simulink library "mySLLib"  (R2025a)
settings: Solver=VariableStepAuto  StartTime=0.0  StopTime=10.0  RelTol=1e-3
undefined symbols (not defined in the file or in its folder): ctrl_KPi, ctrl_Tsample
libraries: simulink x1, libKollege x1
settings Model: Creator=jonat  LastModifiedBy=jonat

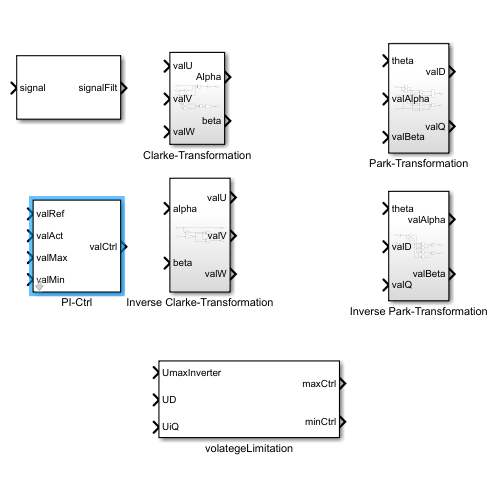
[thumbnail: Simulink's stored preview of the top-level diagram]
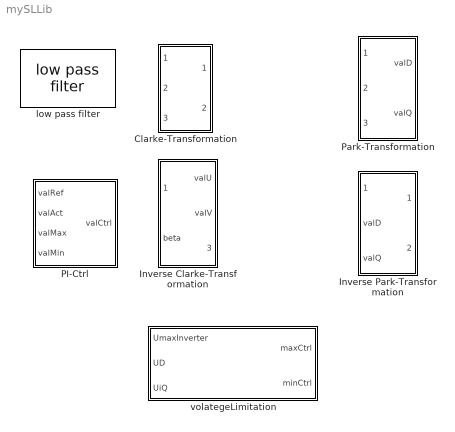
== system mySLLib ==
  Clarke-Transformation : Subsystem
  Inverse Clarke-Transformation : Subsystem
  Inverse Park-Transformation : Subsystem
  PI-Ctrl : Subsystem  mask{localGain=ctrl_KPi, localTsample=ctrl_Tsample, localKi=0}
      mask prompts: localGain "Proportionalfaktor Kp"; localTsample "Abtastzeit (s)"; localKi "Intergralfaktor Ki"
      mask help: Dieser Block implementiert einen zeitdiskreten PI-Regler mit Anti-Wind-up-Funktionalitaet.
      mask DialogControl ParameterGroupVar Prompt: Reglerparameter
  Park-Transformation : Subsystem
  low pass filter : libKollege/low pass filter  localTFilt=1  localTsample=1
  volategeLimitation : Subsystem
      mask help: Berechnung der maximalen Q-Spannung aufgrund der begrenzten Umrichterausgangsspannung.

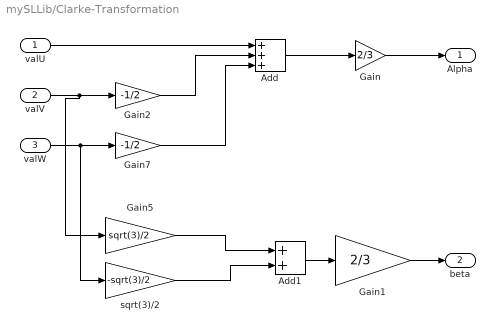
== system mySLLib/Clarke-Transformation ==
  valU : Inport
  valV : Inport  Port=2
  valW : Inport  Port=3
  Add : Sum  Inputs=+++
  Add1 : Sum
  Gain : Gain  Gain=2/3  OutDataTypeStr=single
  Gain1 : Gain  Gain=2/3  OutDataTypeStr=single
  Gain2 : Gain  Gain=-1/2
  Gain5 : Gain  Gain=sqrt(3)/2
  Gain7 : Gain  Gain=-1/2
  sqrt(3)/2 : Gain  Gain=-sqrt(3)/2
  Alpha : Outport
  beta : Outport  Port=2
  wires:
  Gain2/1 -> Add/2
  Gain5/1 -> Add1/1
  Gain1/1 -> beta/1
  sqrt(3)/2/1 -> Add1/2
  Add1/1 -> Gain1/1
  Gain7/1 -> Add/3
  Gain/1 -> Alpha/1
  valU/1 -> Add/1
  valW/1 -> sqrt(3)/2/1, Gain7/1
  Add/1 -> Gain/1
  valV/1 -> Gain2/1, Gain5/1

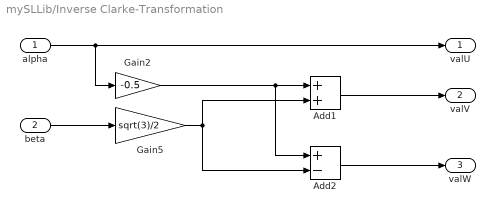
== system mySLLib/Inverse Clarke-Transformation ==
  alpha : Inport
  beta : Inport  Port=2
  Add1 : Sum
  Add2 : Sum  Inputs=+-
  Gain2 : Gain  Gain=-0.5
  Gain5 : Gain  Gain=sqrt(3)/2
  valU : Outport
  valV : Outport  Port=2
  valW : Outport  Port=3
  wires:
  Gain5/1 -> Add2/2, Add1/2
  Add2/1 -> valW/1
  Add1/1 -> valV/1
  Gain2/1 -> Add2/1, Add1/1
  beta/1 -> Gain5/1
  alpha/1 -> valU/1, Gain2/1

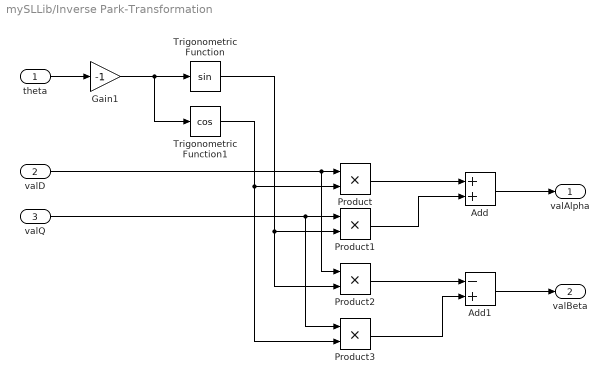
== system mySLLib/Inverse Park-Transformation ==
  theta : Inport
  valD : Inport  Port=2
  valQ : Inport  Port=3
  Add : Sum
  Add1 : Sum  Inputs=-+
  Gain1 : Gain  Gain=-1
  Product{,1..3} (4 alike) : Product
  Trigonometric Function : Trigonometry  OutputSignalType=real
  Trigonometric Function1 : Trigonometry  Operator=cos  OutputSignalType=real
  valAlpha : Outport
  valBeta : Outport  Port=2
  wires:
  Product3/1 -> Add1/2
  Product2/1 -> Add1/1
  Trigonometric Function/1 -> Product1/2, Product2/2
  Product1/1 -> Add/2
  Product/1 -> Add/1
  valQ/1 -> Product3/1, Product1/1
  Trigonometric Function1/1 -> Product/2, Product3/2
  valD/1 -> Product/1, Product2/1
  Gain1/1 -> Trigonometric Function/1, Trigonometric Function1/1
  Add1/1 -> valBeta/1
  Add/1 -> valAlpha/1
  theta/1 -> Gain1/1

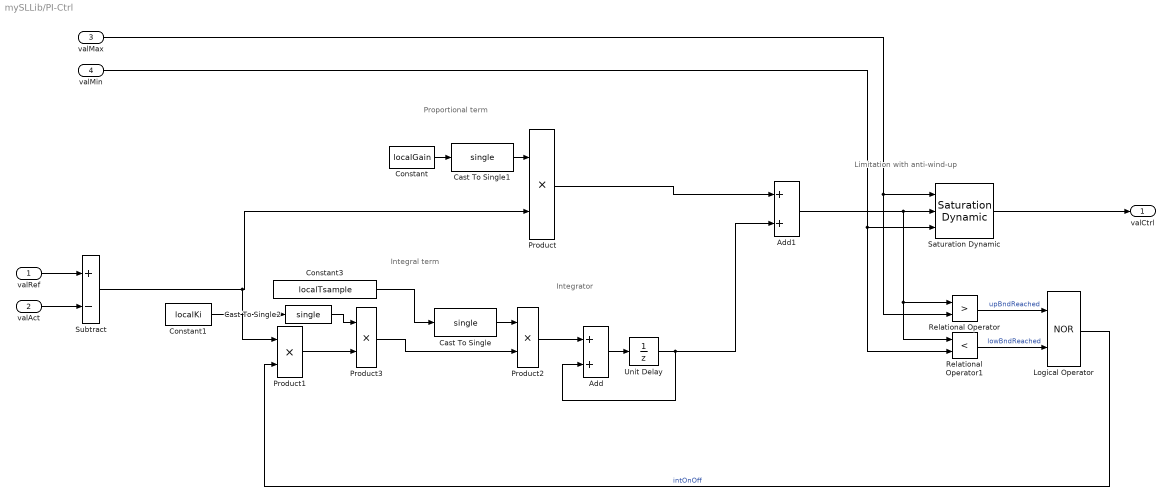
== system mySLLib/PI-Ctrl ==
  note: Integral term
  note: Integrator
  note: Limitation with anti-wind-up
  note: Proportional term
  valRef : Inport
  valAct : Inport  Port=2
  valMax : Inport  Port=3
  valMin : Inport  Port=4
  Add : Sum
  Add1 : Sum
  Cast To Single : DataTypeConversion  OutDataTypeStr=single  SaturateOnIntegerOverflow=off  RndMeth=Floor
  Cast To Single1 : DataTypeConversion  OutDataTypeStr=single  SaturateOnIntegerOverflow=off  RndMeth=Floor
  Cast To Single2 : DataTypeConversion  OutDataTypeStr=single  SaturateOnIntegerOverflow=off  RndMeth=Floor
  Constant : Constant  Value=localGain
  Constant1 : Constant  Value=localKi
  Constant3 : Constant  Value=localTsample
  Logical Operator : Logic  Operator=NOR  AllPortsSameDT=off  OutDataTypeStr=boolean
  Product{,1..3} (4 alike) : Product
  Relational Operator : RelationalOperator  Operator=>  OutDataTypeStr=boolean  InputSameDT=off
  Relational Operator1 : RelationalOperator  Operator=<  OutDataTypeStr=boolean  InputSameDT=off
  Saturation Dynamic : simulink/Discontinuities/Saturation Dynamic  OutMin=[]  OutMax=[]  OutDataTypeStr=Inherit: Same as second input  OutDataType=fixdt(1, 16)  OutScaling=2^-10  DoSatur=off
  Subtract : Sum  Inputs=+-
  Unit Delay : UnitDelay  SampleTime=-1  HasFrameUpgradeWarning=on
  valCtrl : Outport
  wires:
  Add/1 -> Unit Delay/1
  valMin/1 -> Relational Operator1/2, Saturation Dynamic/3
  Logical Operator/1 -> Product1/2  "intOnOff"
  Add1/1 -> Saturation Dynamic/2, Relational Operator/1, Relational Operator1/1
  Product/1 -> Add1/1
  Relational Operator1/1 -> Logical Operator/2  "lowBndReached"
  Constant3/1 -> Cast To Single/1
  valMax/1 -> Saturation Dynamic/1, Relational Operator/2
  Product1/1 -> Product3/2
  Constant/1 -> Cast To Single1/1
  Saturation Dynamic/1 -> valCtrl/1
  valAct/1 -> Subtract/2
  Relational Operator/1 -> Logical Operator/1  "upBndReached"
  Subtract/1 -> Product1/1, Product/2
  valRef/1 -> Subtract/1
  Unit Delay/1 -> Add/2, Add1/2
  Product2/1 -> Add/1
  Cast To Single/1 -> Product2/1
  Cast To Single1/1 -> Product/1
  Product3/1 -> Product2/2
  Cast To Single2/1 -> Product3/1
  Constant1/1 -> Cast To Single2/1

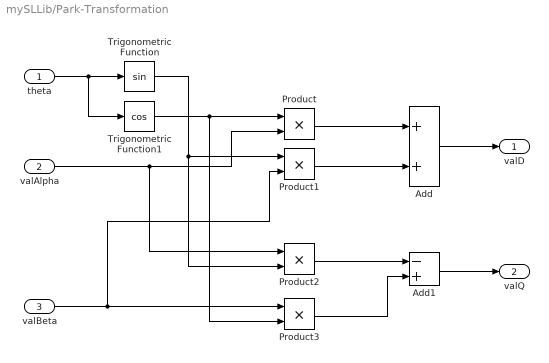
== system mySLLib/Park-Transformation ==
  theta : Inport
  valAlpha : Inport  Port=2
  valBeta : Inport  Port=3
  Add : Sum
  Add1 : Sum  Inputs=-+
  Product{,1..3} (4 alike) : Product
  Trigonometric Function : Trigonometry  OutputSignalType=real
  Trigonometric Function1 : Trigonometry  Operator=cos  OutputSignalType=real
  valD : Outport
  valQ : Outport  Port=2
  wires:
  Product3/1 -> Add1/2
  Product2/1 -> Add1/1
  Trigonometric Function/1 -> Product2/2, Product1/1
  Product/1 -> Add/1
  Product1/1 -> Add/2
  valBeta/1 -> Product1/2, Product3/1
  Trigonometric Function1/1 -> Product3/2, Product/1
  valAlpha/1 -> Product/2, Product2/1
  theta/1 -> Trigonometric Function1/1, Trigonometric Function/1
  Add/1 -> valD/1
  Add1/1 -> valQ/1

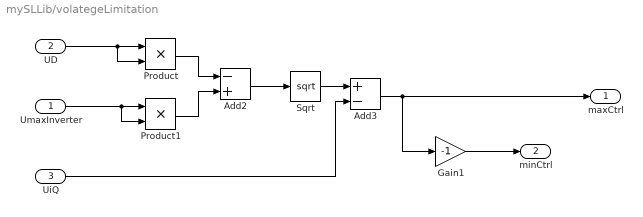
== system mySLLib/volategeLimitation ==
  UmaxInverter : Inport
  UD : Inport  Port=2
  UiQ : Inport  Port=3
  Add2 : Sum  Inputs=-+
  Add3 : Sum  Inputs=+-
  Gain1 : Gain  Gain=-1
  Product : Product
  Product1 : Product
  Sqrt : Sqrt
  maxCtrl : Outport
  minCtrl : Outport  Port=2
  wires:
  Add2/1 -> Sqrt/1
  UmaxInverter/1 -> Product1/1, Product1/2
  Product/1 -> Add2/1
  Add3/1 -> maxCtrl/1, Gain1/1
  Product1/1 -> Add2/2
  Gain1/1 -> minCtrl/1
  UD/1 -> Product/2, Product/1
  UiQ/1 -> Add3/2
  Sqrt/1 -> Add3/1
